simulink library "LCDScope"  (R2015a)
settings: Solver=ode45  StartTime=0.0  StopTime=10.0  RelTol=1e-3
libraries: mbed_lib x1
settings Model: CovSFcnEnable=off  Creator=Schlueter  LastModifiedBy=Stuv
settings DebuggingCC: SolverPrmCheckMsg=warning

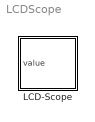
== system LCDScope ==
  LCD-Scope : Subsystem  mask(LCD-Scope){MinValue=0, MaxValue=120, StepSize=1, TimeRange=500, scaleValue=1e0}
      mask prompts: MinValue "Min Value"; MaxValue "Max Value"; StepSize "Step Size"; TimeRange "Samples per Window"; scaleValue "Scale Value"
      mask help:
      | Dieser Block kann genutzt werden um Signale mit dem LCD Mi0283QT darzustellen.
      | Für die Kommunikation wird SPI verwendet. Die verwendeten PINs lassen sich innerhalb des Blocks einstellen und ändern.
      mask init:
      | StepSize = 1;
      mask Display: disp('Scope')

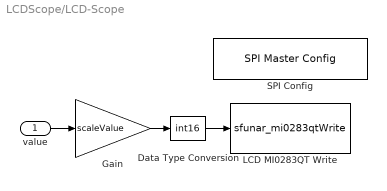
== system LCDScope/LCD-Scope ==
  value : Inport
  Data Type Conversion : DataTypeConversion  OutDataTypeStr=int16
  Gain : Gain  Gain=scaleValue
  LCD MI0283QT Write : S-Function  FunctionName=sfunar_mi0283qtWrite  Parameters=int16(MinValue), int16(MaxValue), uint16(StepSize), uint16(TimeRange), int8(SPIPort), uint8(CSPort), uint8(CSPin), uint8(RSTPort), uint8(RSTPin)  mask(Draw Value on LCD-Scope){SPIPort=1, CSPort=B, CSPin=11, RSTPort=B, RSTPin=10, MinValue=MinValue*scaleValue, MaxValue=MaxValue*scaleValue, StepSize=StepSize, TimeRange=TimeRange}
      mask prompts: SPIPort "SPI Port"; CSPort "CS: Port"; CSPin "Pin"; RSTPort "RST: Port"; RSTPin "Pin"; MinValue "Min Value"; MaxValue "Max Value"; StepSize "Step Size"; TimeRange "Time Range"
      mask TypeOptions SPIPort: 1 | 2 | 3 | 4
      mask TypeOptions CSPort: A | B | C | D | E | F
      mask TypeOptions CSPin: 0 | 1 | 2 | 3 | 4 | 5 | 6 | 7 | 8 | 9 | 10 | 11 | 12 | 13 | 14 | 15
      mask TypeOptions RSTPort: A | B | C | D | E | F
      mask TypeOptions RSTPin: 0 | 1 | 2 | 3 | 4 | 5 | 6 | 7 | 8 | 9 | 10 | 11 | 12 | 13 | 14 | 15
      mask Display:
      | disp(['Write Scope' ' \n\n']);
      | disp(['\n\nSPI ' num2str(SPIPort) '\n']);
      | disp(['\n\n\n\nCS: ' CSPort+64 '.' num2str(CSPin-1) ', RST: ' RSTPort+64, '.' num2str(RSTPin-1) ' \n']);
  SPI Config : mbed_lib/SPI/SPI Master Config  Priority=0  SpiPort=1  SParameter6=8000000  SParameter2=B  SParameter3=5  SParameter4=B  SParameter5=4  SCK_PORT=B  SCK_PIN=3
  wires:
  value/1 -> Gain/1
  Data Type Conversion/1 -> LCD MI0283QT Write/1
  Gain/1 -> Data Type Conversion/1
